simulink model "gm_sampleModel1971_sub"  (R2023a)
settings: Solver=VariableStepAuto  StartTime=0.0  StopTime=10.0  RelTol=1e-3
libraries: hdlsllib x1, simulink x1
settings Model: Creator=user1  LastModifiedBy=user1
settings OptimizationCC: BlockReduction=off  ConditionallyExecuteInputs=off
settings DebuggingCC: InheritedTsInSrcMsg=none

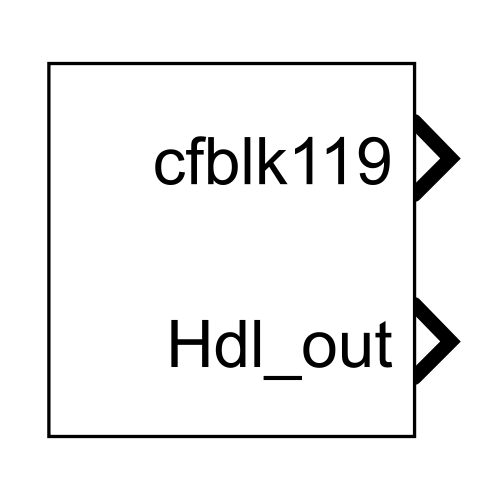
[thumbnail: Simulink's stored preview of the top-level diagram]
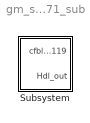
== system gm_sampleModel1971_sub ==
  Subsystem : Subsystem

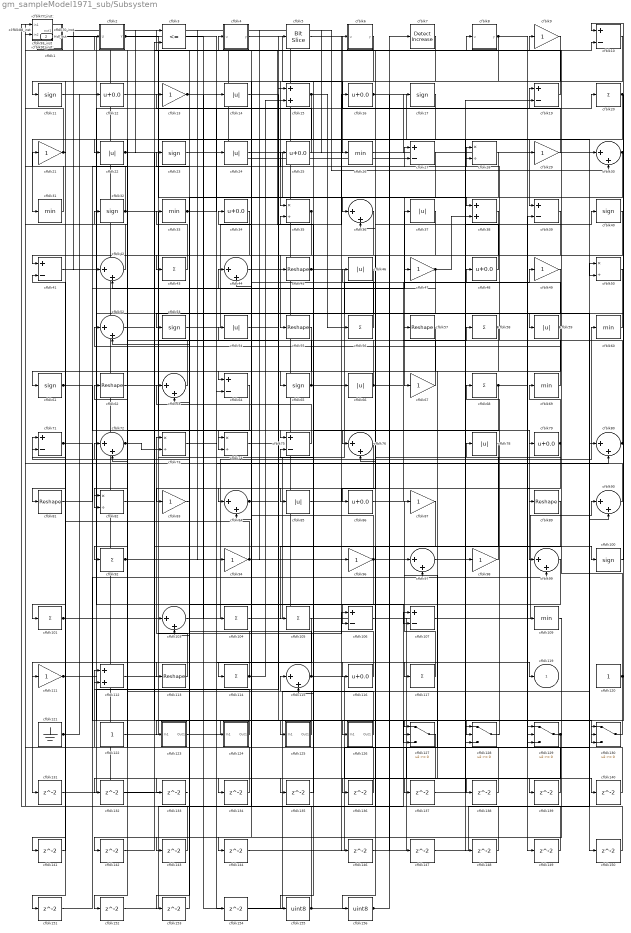
== system gm_sampleModel1971_sub/Subsystem ==
  cfblk1 : Subsystem  mask(Detect Fall Negative){vinit=double(0), InputProcessing=Elements as channels (sample based), OutDataTypeStr=uint8}
      mask prompts: vinit "Simulink:masks:InitialCondition_MP"; InputProcessing "Simulink:masks:InputProcessing_MP"; OutDataTypeStr "Simulink:masks:OutputDataType_MP"
      mask help: Simulink:masks:DetectFallNegative_MD
      mask init:
      | InputProcessing = 'Elements as channels (sample based)';
      | OutDataTypeStr = 'uint8';
      | vinit = double(0);
      mask TypeOptions InputProcessing: Simulink:masks:ColumnsAsChannelsFrameBased | Simulink:masks:ElementsAsChannelsSampleBased
      mask TypeOptions OutDataTypeStr: Simulink:masks:uint8 | Simulink:masks:boolean
      mask Display: fprintf('U < 0\n&  NOT\nU/z < 0')
  cfblk{10,19,27,39,41,64,71,75,106..107} (10 alike) : Sum  Inputs=+-  OutDataTypeStr=uint8
  cfblk{11,17,23,32,40,53,61,65,100} (9 alike) : Signum
  cfblk{20,43,56,58,68,92,101,104..105,114,117} (11 alike) : Sum  Inputs=+  OutDataTypeStr=uint8
  cfblk102_inst : Subsystem
  cfblk{30,36,42,44,52,63,72,76,80,84,90,97,99,103,115} (15 alike) : Sum  Inputs=|++  OutDataTypeStr=uint8
  cfblk108_inst : Subsystem
  cfblk{26,31,33,60,69,109} (6 alike) : MinMax  OutDataTypeStr=uint8
  cfblk110_inst : Subsystem
  cfblk{9,13,21,29,47,49,67,83,87,94,96,98,111} (13 alike) : Gain  OutDataTypeStr=uint8
  cfblk112 : Sum  OutDataTypeStr=uint8
  cfblk{45,55,57,62,81,89,113} (7 alike) : Reshape
  cfblk{12,16,25,34,48,79,86,116} (8 alike) : Bias  Bias=0.0  SaturateOnIntegerOverflow=off
  cfblk120 : Constant  OutDataTypeStr=uint8  SampleTime=-1
  cfblk121 : Ground
  cfblk122 : Constant  OutDataTypeStr=uint8  SampleTime=-1
  cfblk123 : Subsystem
  cfblk124 : Subsystem
  cfblk125 : Subsystem
  cfblk126 : Subsystem
  cfblk{127..130} (4 alike) : Switch  OutDataTypeStr=uint8  SaturateOnIntegerOverflow=off  InputSameDT=off
  cfblk{131..144,146..154} (23 alike) : Delay  SampleTime=1
  cfblk{14,22,24,37,46,54,59,66,78,85} (10 alike) : Abs  OutDataTypeStr=uint8  SaturateOnIntegerOverflow=off
  cfblk15 : Sum  OutDataTypeStr=uint8
  cfblk155 : DataTypeConversion  OutDataTypeStr=uint8  SaturateOnIntegerOverflow=off  RndMeth=Floor
  cfblk156 : DataTypeConversion  OutDataTypeStr=uint8  SaturateOnIntegerOverflow=off  RndMeth=Floor
  cfblk18_inst : Subsystem
  cfblk2 : Subsystem  mask(Detect Fall Nonpositive){vinit=double(0), InputProcessing=Elements as channels (sample based), OutDataTypeStr=uint8}
      mask prompts: vinit "Simulink:masks:InitialCondition_MP"; InputProcessing "Simulink:masks:InputProcessing_MP"; OutDataTypeStr "Simulink:masks:OutputDataType_MP"
      mask help: Simulink:masks:DetectFallNonpositive_MD
      mask init:
      | InputProcessing = 'Elements as channels (sample based)';
      | OutDataTypeStr = 'uint8';
      | vinit = double(0);
      mask TypeOptions InputProcessing: Simulink:masks:ColumnsAsChannelsFrameBased | Simulink:masks:ElementsAsChannelsSampleBased
      mask TypeOptions OutDataTypeStr: Simulink:masks:uint8 | Simulink:masks:boolean
      mask Display: fprintf('U <= 0\n&  NOT\nU/z <= 0')
  cfblk{28,35,50,73..74,82} (6 alike) : Product  Inputs=*/  OutDataTypeStr=uint8  RndMeth=Zero  SaturateOnIntegerOverflow=on
  cfblk3 : RelationalOperator  Operator=<=  OutDataTypeStr=boolean  InputSameDT=off
  cfblk38 : Sum  OutDataTypeStr=uint8
  cfblk4 : Subsystem  mask(Compare To Zero){relop=<=, OutDataTypeStr=uint8, ZeroCross=on}
      mask prompts: relop "Simulink:masks:Operator_MP"; OutDataTypeStr "Simulink:masks:OutputDataType_MP"; ZeroCross "Simulink:masks:EnableZerocrossingDetection_MP"
      mask help: Simulink:masks:CompareToZero_MD
      mask init:
      | OutDataTypeStr = 'uint8';
      | ZeroCross = 'on';
      | blkName = 'sampleModel1971_sub/Subsystem/cfblk4';
      | relop = '<=';
      | setValue = 'fixdt(0, 8)';
      mask TypeOptions relop: == | ~= | < | <= | >= | >
      mask TypeOptions OutDataTypeStr: Simulink:masks:uint8 | Simulink:masks:boolean
      mask Callback ZeroCross: sl('zeroCrossEnable', gcbh);
      mask Display: disp([relop,' 0'])
  cfblk5 : hdlsllib/Logic and Bit Operations/Bit Slice  lidx=7  ridx=0
  cfblk6 : Subsystem  mask(Compare To Zero){relop=<=, OutDataTypeStr=uint8, ZeroCross=on}
      mask prompts: relop "Simulink:masks:Operator_MP"; OutDataTypeStr "Simulink:masks:OutputDataType_MP"; ZeroCross "Simulink:masks:EnableZerocrossingDetection_MP"
      mask help: Simulink:masks:CompareToZero_MD
      mask init:
      | OutDataTypeStr = 'uint8';
      | ZeroCross = 'on';
      | blkName = 'sampleModel1971_sub/Subsystem/cfblk6';
      | relop = '<=';
      | setValue = 'fixdt(0, 8)';
      mask TypeOptions relop: == | ~= | < | <= | >= | >
      mask TypeOptions OutDataTypeStr: Simulink:masks:uint8 | Simulink:masks:boolean
      mask Callback ZeroCross: sl('zeroCrossEnable', gcbh);
      mask Display: disp([relop,' 0'])
  cfblk7 : simulink/Logic and Bit Operations/Detect Increase  vinit=0.0  OutDataTypeStr=uint8
      settings: LibrarySourceBlock=|
      | hdlsllib/Logic and Bit
      | Operations/Detect
      | Increase
  cfblk70_inst : Subsystem
  cfblk77_inst : Subsystem
  cfblk8 : Subsystem  mask(Compare To Zero){relop=<=, OutDataTypeStr=uint8, ZeroCross=on}
      mask prompts: relop "Simulink:masks:Operator_MP"; OutDataTypeStr "Simulink:masks:OutputDataType_MP"; ZeroCross "Simulink:masks:EnableZerocrossingDetection_MP"
      mask help: Simulink:masks:CompareToZero_MD
      mask init:
      | OutDataTypeStr = 'uint8';
      | ZeroCross = 'on';
      | blkName = 'sampleModel1971_sub/Subsystem/cfblk8';
      | relop = '<=';
      | setValue = 'fixdt(0, 8)';
      mask TypeOptions relop: == | ~= | < | <= | >= | >
      mask TypeOptions OutDataTypeStr: Simulink:masks:uint8 | Simulink:masks:boolean
      mask Callback ZeroCross: sl('zeroCrossEnable', gcbh);
      mask Display: disp([relop,' 0'])
  cfblk88_inst : Subsystem
  cfblk91_inst : Subsystem
  cfblk93_inst : Subsystem
  cfblk119 : Outport  OutDataTypeStr=uint8  SampleTime=1  VectorParamsAs1DForOutWhenUnconnected=off
  Hdl_out : Outport  Port=2  OutDataTypeStr=uint8  SampleTime=1
  wires:
  cfblk1/1(Y) -> cfblk75/1
  cfblk10/1 -> cfblk35/1
  cfblk100/1 -> cfblk10/1
  cfblk101/1 -> cfblk10/2, cfblk8/1(u)
  cfblk102_inst/1(out1) -> cfblk88_inst/2(in2), cfblk14/1
  cfblk103/1 -> cfblk60/1
  cfblk104/1 -> cfblk49/1
  cfblk105/1 -> cfblk131/1
  cfblk106/1 -> cfblk139/1
  cfblk107/1 -> cfblk90/1
  cfblk108_inst/1(out1) -> cfblk24/1
  cfblk109/1 -> cfblk142/1
  cfblk11/1 -> cfblk106/2
  cfblk110_inst/1(out1) -> cfblk96/1
  cfblk111/1 -> cfblk19/1, cfblk130/3
  cfblk112/1 -> cfblk94/1
  cfblk113/1 -> cfblk73/1
  cfblk114/1 -> cfblk72/1, cfblk15/2
  cfblk115/1 -> cfblk71/1, cfblk52/2, cfblk138/1
  cfblk116/1 -> cfblk35/2
  cfblk117/1 -> cfblk87/1
  cfblk12/1 -> cfblk38/1
  cfblk120/1 -> cfblk78/1, cfblk70_inst/2(in2), cfblk52/1, cfblk127/1
  cfblk121/1 -> cfblk91_inst/1(in1), cfblk12/1
  cfblk122/1 -> cfblk106/1
  cfblk123/1(Out1) -> cfblk128/2
  cfblk124/1(Out1) -> cfblk112/1
  cfblk125/1(Out1) -> cfblk62/1
  cfblk126/1(Out1) -> cfblk115/1
  cfblk127/1 -> cfblk152/1
  cfblk128/1 -> cfblk68/1
  cfblk129/1 -> cfblk134/1, cfblk133/1
  cfblk13/1 -> cfblk127/2, cfblk104/1
  cfblk130/1 -> cfblk123/1(In1)
  cfblk131/1 -> cfblk27/1
  cfblk132/1 -> cfblk28/1
  cfblk133/1 -> cfblk1/1(U)
  cfblk134/1 -> cfblk108_inst/2(in2)
  cfblk135/1 -> cfblk75/2
  cfblk136/1 -> cfblk72/2
  cfblk137/1 -> cfblk19/2
  cfblk138/1 -> cfblk77_inst/2(in2)
  cfblk139/1 -> cfblk97/1
  cfblk14/1 -> cfblk126/1(In1)
  cfblk140/1 -> cfblk112/2
  cfblk141/1 -> cfblk71/2
  cfblk142/1 -> cfblk103/1
  cfblk143/1 -> cfblk18_inst/1(in1)
  cfblk144/1 -> cfblk39/2
  cfblk146/1 -> cfblk90/2
  cfblk147/1 -> cfblk50/1
  cfblk148/1 -> cfblk93_inst/2(in2)
  cfblk149/1 -> cfblk44/2
  cfblk15/1 -> cfblk22/1, cfblk92/1, cfblk56/1
  cfblk150/1 -> cfblk36/2
  cfblk151/1 -> cfblk99/2
  cfblk152/1 -> cfblk107/1
  cfblk153/1 -> cfblk63/2
  cfblk154/1 -> cfblk80/1
  cfblk155/1 -> cfblk34/1, cfblk23/1
  cfblk156/1 -> Hdl_out/1, cfblk7/1
  cfblk16/1 -> cfblk129/2, cfblk148/1, cfblk147/1
  cfblk17/1 -> cfblk101/1
  cfblk18_inst/1(out1) -> cfblk30/2
  cfblk19/1 -> cfblk18_inst/2(in2)
  cfblk2/1(Y) -> cfblk39/1, cfblk50/2
  cfblk20/1 -> cfblk130/2, cfblk74/2, cfblk31/1
  cfblk21/1 -> cfblk91_inst/2(in2), cfblk61/1
  cfblk22/1 -> cfblk100/1, cfblk9/1
  cfblk23/1 -> cfblk116/1
  cfblk24/1 -> cfblk66/1
  cfblk25/1 -> cfblk4/1(u)
  cfblk26/1 -> cfblk17/1
  cfblk27/1 -> cfblk36/1
  cfblk28/1 -> cfblk67/1
  cfblk29/1 -> cfblk6/1(u)
  cfblk3/1 -> cfblk124/1(In1)
  cfblk30/1 -> cfblk85/1, cfblk83/1
  cfblk31/1 -> cfblk110_inst/1(in1)
  cfblk32/1 -> cfblk99/1, cfblk102_inst/2(in2)
  cfblk33/1 -> cfblk64/2, cfblk20/1
  cfblk34/1 -> cfblk43/1
  cfblk35/1 -> cfblk84/2, cfblk141/1
  cfblk36/1 -> cfblk114/1
  cfblk37/1 -> cfblk86/1
  cfblk38/1 -> cfblk82/2
  cfblk39/1 -> cfblk55/1
  cfblk4/1(y) -> cfblk26/1
  cfblk40/1 -> cfblk81/1
  cfblk41/1 -> cfblk59/1
  cfblk42/1 -> cfblk88_inst/1(in1)
  cfblk43/1 -> cfblk33/1
  cfblk44/1 -> cfblk5/1
  cfblk45/1 -> cfblk150/1, cfblk149/1
  cfblk46/1 -> cfblk65/1
  cfblk47/1 -> cfblk76/2, cfblk42/2, cfblk38/2, cfblk115/2
  cfblk48/1 -> cfblk77_inst/1(in1)
  cfblk49/1 -> cfblk153/1
  cfblk5/1 -> cfblk107/2
  cfblk50/1 -> cfblk53/1
  cfblk52/1 -> cfblk79/1
  cfblk53/1 -> cfblk16/1
  cfblk54/1 -> cfblk76/1
  cfblk55/1 -> cfblk111/1
  cfblk56/1 -> cfblk102_inst/1(in1)
  cfblk57/1 -> cfblk113/1
  cfblk58/1 -> cfblk84/1, cfblk137/1
  cfblk59/1 -> cfblk64/1, cfblk37/1, cfblk82/1
  cfblk6/1(y) -> cfblk144/1
  cfblk60/1 -> cfblk57/1
  cfblk61/1 -> cfblk74/1, cfblk151/1
  cfblk62/1 -> cfblk15/1
  cfblk63/1 -> cfblk93_inst/1(in1)
  cfblk64/1 -> cfblk132/1
  cfblk65/1 -> cfblk127/3, cfblk21/1
  cfblk66/1 -> cfblk54/1, cfblk48/1, cfblk46/1
  cfblk67/1 -> cfblk44/1
  cfblk68/1 -> cfblk129/1, cfblk135/1
  cfblk69/1 -> cfblk70_inst/1(in1)
  cfblk7/1 -> cfblk155/1
  cfblk70_inst/1(out1) -> cfblk109/1
  cfblk71/1 -> cfblk25/1, cfblk128/3
  cfblk72/1 -> cfblk32/1, cfblk73/2
  cfblk73/1 -> cfblk80/2
  cfblk74/1 -> cfblk45/1
  cfblk75/1 -> cfblk63/1
  cfblk76/1 -> cfblk143/1
  cfblk77_inst/1(out1) -> cfblk98/1
  cfblk78/1 -> cfblk156/1
  cfblk79/1 -> cfblk129/3, cfblk69/1
  cfblk8/1(y) -> cfblk130/1, cfblk11/1, cfblk140/1
  cfblk80/1 -> cfblk110_inst/2(in2), cfblk28/2
  cfblk81/1 -> cfblk47/1
  cfblk82/1 -> cfblk128/1
  cfblk83/1 -> cfblk3/1
  cfblk84/1 -> cfblk119/1, cfblk117/1
  cfblk85/1 -> cfblk89/1
  cfblk86/1 -> cfblk58/1
  cfblk87/1 -> cfblk136/1
  cfblk88_inst/1(out1) -> cfblk29/1
  cfblk89/1 -> cfblk105/1
  cfblk9/1 -> cfblk41/1
  cfblk90/1 -> cfblk108_inst/1(in1)
  cfblk91_inst/1(out1) -> cfblk30/1
  cfblk92/1 -> cfblk3/2, cfblk154/1
  cfblk93_inst/1(out1) -> cfblk42/1, cfblk27/2
  cfblk94/1 -> cfblk97/2, cfblk41/2, cfblk146/1
  cfblk96/1 -> cfblk13/1, cfblk125/1(In1)
  cfblk97/1 -> cfblk40/1
  cfblk98/1 -> cfblk2/1(U)
  cfblk99/1 -> cfblk103/2

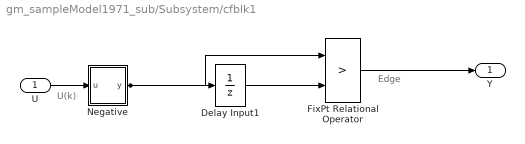
== system gm_sampleModel1971_sub/Subsystem/cfblk1 ==
  note: U(k)
  note: Edge
  U : Inport  OutDataTypeStr=uint8  SampleTime=1
  Delay Input1 : UnitDelay  Description=Store in Global RAM  DisableCoverage=on  InitialCondition=vinit  SampleTime=-1  HasFrameUpgradeWarning=on
  FixPt Relational Operator : RelationalOperator  Operator=>  OutDataTypeStr=fixdt(0, 8)  ZeroCross=off  InputSameDT=off
  Negative : Subsystem  mask(Compare To Zero){relop=<, OutDataTypeStr=boolean, ZeroCross=off}
      mask prompts: relop "Simulink:masks:Operator_MP"; OutDataTypeStr "Simulink:masks:OutputDataType_MP"; ZeroCross "Simulink:masks:EnableZerocrossingDetection_MP"
      mask help: Simulink:masks:CompareToZero_MD
      mask init:
      | OutDataTypeStr = 'boolean';
      | ZeroCross = 'off';
      | blkName = 'sampleModel1971_sub/Subsystem/cfblk1/Negative';
      | relop = '<';
      | setValue = 'boolean';
      mask TypeOptions relop: == | ~= | < | <= | >= | >
      mask TypeOptions OutDataTypeStr: Simulink:masks:uint8 | Simulink:masks:boolean
      mask Callback ZeroCross: sl('zeroCrossEnable', gcbh);
      mask Display: disp([relop,' 0'])
  Y : Outport  SampleTime=1
  wires:
  U/1 -> Negative/1(u)
  Delay Input1/1 -> FixPt Relational Operator/2
  FixPt Relational Operator/1 -> Y/1
  Negative/1(y) -> FixPt Relational Operator/1, Delay Input1/1

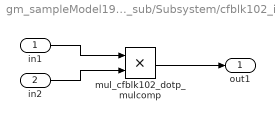
== system gm_sampleModel1971_sub/Subsystem/cfblk102_inst ==
  in1 : Inport  OutDataTypeStr=uint8  SampleTime=1
  in2 : Inport  Port=2  OutDataTypeStr=uint8  SampleTime=1
  mul_cfblk102_dotp_mulcomp : Product  Inputs=**  OutDataTypeStr=uint8  SampleTime=1
  out1 : Outport  OutDataTypeStr=uint8  SampleTime=1
  wires:
  in1/1 -> mul_cfblk102_dotp_mulcomp/1
  in2/1 -> mul_cfblk102_dotp_mulcomp/2
  mul_cfblk102_dotp_mulcomp/1 -> out1/1

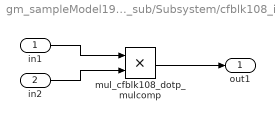
== system gm_sampleModel1971_sub/Subsystem/cfblk108_inst ==
  in1 : Inport  OutDataTypeStr=uint8  SampleTime=1
  in2 : Inport  Port=2  OutDataTypeStr=uint8  SampleTime=1
  mul_cfblk108_dotp_mulcomp : Product  Inputs=**  OutDataTypeStr=uint8  SampleTime=1
  out1 : Outport  OutDataTypeStr=uint8  SampleTime=1
  wires:
  in1/1 -> mul_cfblk108_dotp_mulcomp/1
  in2/1 -> mul_cfblk108_dotp_mulcomp/2
  mul_cfblk108_dotp_mulcomp/1 -> out1/1

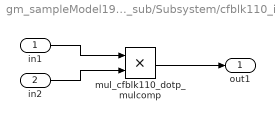
== system gm_sampleModel1971_sub/Subsystem/cfblk110_inst ==
  in1 : Inport  OutDataTypeStr=uint8  SampleTime=1
  in2 : Inport  Port=2  OutDataTypeStr=uint8  SampleTime=1
  mul_cfblk110_dotp_mulcomp : Product  Inputs=**  OutDataTypeStr=uint8  SampleTime=1
  out1 : Outport  OutDataTypeStr=uint8  SampleTime=1
  wires:
  in1/1 -> mul_cfblk110_dotp_mulcomp/1
  in2/1 -> mul_cfblk110_dotp_mulcomp/2
  mul_cfblk110_dotp_mulcomp/1 -> out1/1

== system gm_sampleModel1971_sub/Subsystem/cfblk123 ==
  In1 : Inport  OutDataTypeStr=uint8  PortDimensions=1  SampleTime=1
  Out1 : Outport  SampleTime=1
  wires:
  In1/1 -> Out1/1

== system gm_sampleModel1971_sub/Subsystem/cfblk124 ==
  In1 : Inport  OutDataTypeStr=boolean  PortDimensions=1  SampleTime=1
  Out1 : Outport  SampleTime=1
  wires:
  In1/1 -> Out1/1

== system gm_sampleModel1971_sub/Subsystem/cfblk125 ==
  In1 : Inport  OutDataTypeStr=uint8  PortDimensions=1  SampleTime=1
  Out1 : Outport  SampleTime=1
  wires:
  In1/1 -> Out1/1

== system gm_sampleModel1971_sub/Subsystem/cfblk126 ==
  In1 : Inport  OutDataTypeStr=uint8  PortDimensions=1  SampleTime=1
  Out1 : Outport  SampleTime=1
  wires:
  In1/1 -> Out1/1

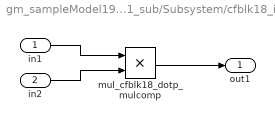
== system gm_sampleModel1971_sub/Subsystem/cfblk18_inst ==
  in1 : Inport  OutDataTypeStr=uint8  SampleTime=1
  in2 : Inport  Port=2  OutDataTypeStr=uint8  SampleTime=1
  mul_cfblk18_dotp_mulcomp : Product  Inputs=**  OutDataTypeStr=uint8  SampleTime=1
  out1 : Outport  OutDataTypeStr=uint8  SampleTime=1
  wires:
  in1/1 -> mul_cfblk18_dotp_mulcomp/1
  in2/1 -> mul_cfblk18_dotp_mulcomp/2
  mul_cfblk18_dotp_mulcomp/1 -> out1/1

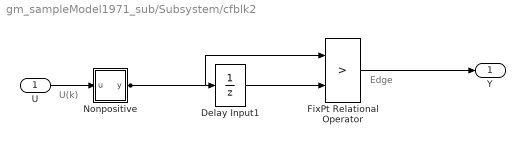
== system gm_sampleModel1971_sub/Subsystem/cfblk2 ==
  note: U(k)
  note: Edge
  U : Inport  OutDataTypeStr=uint8  SampleTime=1
  Delay Input1 : UnitDelay  Description=Store in Global RAM  DisableCoverage=on  InitialCondition=vinit  SampleTime=-1  HasFrameUpgradeWarning=on
  FixPt Relational Operator : RelationalOperator  Operator=>  OutDataTypeStr=fixdt(0, 8)  ZeroCross=off  InputSameDT=off
  Nonpositive : Subsystem  mask(Compare To Zero){relop=<=, OutDataTypeStr=boolean, ZeroCross=off}
      mask prompts: relop "Simulink:masks:Operator_MP"; OutDataTypeStr "Simulink:masks:OutputDataType_MP"; ZeroCross "Simulink:masks:EnableZerocrossingDetection_MP"
      mask help: Simulink:masks:CompareToZero_MD
      mask init:
      | OutDataTypeStr = 'boolean';
      | ZeroCross = 'off';
      | blkName = 'sampleModel1971_sub/Subsystem/cfblk2/Nonpositive';
      | relop = '<=';
      | setValue = 'boolean';
      mask TypeOptions relop: == | ~= | < | <= | >= | >
      mask TypeOptions OutDataTypeStr: Simulink:masks:uint8 | Simulink:masks:boolean
      mask Callback ZeroCross: sl('zeroCrossEnable', gcbh);
      mask Display: disp([relop,' 0'])
  Y : Outport  SampleTime=1
  wires:
  U/1 -> Nonpositive/1(u)
  Delay Input1/1 -> FixPt Relational Operator/2
  FixPt Relational Operator/1 -> Y/1
  Nonpositive/1(y) -> FixPt Relational Operator/1, Delay Input1/1

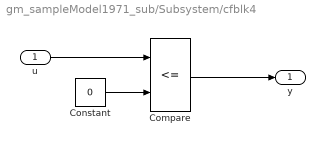
== system gm_sampleModel1971_sub/Subsystem/cfblk4 ==
  u : Inport  OutDataTypeStr=uint8  SampleTime=1
  Compare : RelationalOperator  Operator=<=  OutDataTypeStr=fixdt(0, 8)
  Constant : Constant  DisableCoverage=on  Value=0  OutDataTypeStr=Inherit: Inherit via back propagation  SampleTime=-1  PreserveConstantTs=on
  y : Outport  SampleTime=1
  wires:
  u/1 -> Compare/1
  Compare/1 -> y/1
  Constant/1 -> Compare/2

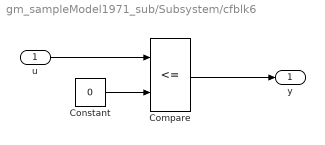
== system gm_sampleModel1971_sub/Subsystem/cfblk6 ==
  u : Inport  OutDataTypeStr=uint8  SampleTime=1
  Compare : RelationalOperator  Operator=<=  OutDataTypeStr=fixdt(0, 8)
  Constant : Constant  DisableCoverage=on  Value=0  OutDataTypeStr=Inherit: Inherit via back propagation  SampleTime=-1  PreserveConstantTs=on
  y : Outport  SampleTime=1
  wires:
  u/1 -> Compare/1
  Compare/1 -> y/1
  Constant/1 -> Compare/2

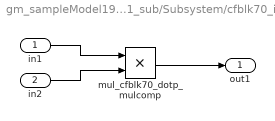
== system gm_sampleModel1971_sub/Subsystem/cfblk70_inst ==
  in1 : Inport  OutDataTypeStr=uint8  SampleTime=1
  in2 : Inport  Port=2  OutDataTypeStr=uint8  SampleTime=1
  mul_cfblk70_dotp_mulcomp : Product  Inputs=**  OutDataTypeStr=uint8  SampleTime=1
  out1 : Outport  OutDataTypeStr=uint8  SampleTime=1
  wires:
  in1/1 -> mul_cfblk70_dotp_mulcomp/1
  in2/1 -> mul_cfblk70_dotp_mulcomp/2
  mul_cfblk70_dotp_mulcomp/1 -> out1/1

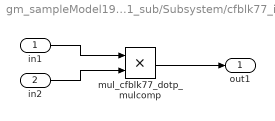
== system gm_sampleModel1971_sub/Subsystem/cfblk77_inst ==
  in1 : Inport  OutDataTypeStr=uint8  SampleTime=1
  in2 : Inport  Port=2  OutDataTypeStr=uint8  SampleTime=1
  mul_cfblk77_dotp_mulcomp : Product  Inputs=**  OutDataTypeStr=uint8  SampleTime=1
  out1 : Outport  OutDataTypeStr=uint8  SampleTime=1
  wires:
  in1/1 -> mul_cfblk77_dotp_mulcomp/1
  in2/1 -> mul_cfblk77_dotp_mulcomp/2
  mul_cfblk77_dotp_mulcomp/1 -> out1/1

== system gm_sampleModel1971_sub/Subsystem/cfblk8 ==
  u : Inport  OutDataTypeStr=uint8  SampleTime=1
  Compare : RelationalOperator  Operator=<=  OutDataTypeStr=fixdt(0, 8)
  Constant : Constant  DisableCoverage=on  Value=0  OutDataTypeStr=Inherit: Inherit via back propagation  SampleTime=-1  PreserveConstantTs=on
  y : Outport  SampleTime=1
  wires:
  u/1 -> Compare/1
  Compare/1 -> y/1
  Constant/1 -> Compare/2

== system gm_sampleModel1971_sub/Subsystem/cfblk88_inst ==
  in1 : Inport  OutDataTypeStr=uint8  SampleTime=1
  in2 : Inport  Port=2  OutDataTypeStr=uint8  SampleTime=1
  mul_cfblk88_dotp_mulcomp : Product  Inputs=**  OutDataTypeStr=uint8  SampleTime=1
  out1 : Outport  OutDataTypeStr=uint8  SampleTime=1
  wires:
  in1/1 -> mul_cfblk88_dotp_mulcomp/1
  in2/1 -> mul_cfblk88_dotp_mulcomp/2
  mul_cfblk88_dotp_mulcomp/1 -> out1/1

== system gm_sampleModel1971_sub/Subsystem/cfblk91_inst ==
  in1 : Inport  OutDataTypeStr=uint8  SampleTime=1
  in2 : Inport  Port=2  OutDataTypeStr=uint8  SampleTime=1
  mul_cfblk91_dotp_mulcomp : Product  Inputs=**  OutDataTypeStr=uint8  SampleTime=1
  out1 : Outport  OutDataTypeStr=uint8  SampleTime=1
  wires:
  in1/1 -> mul_cfblk91_dotp_mulcomp/1
  in2/1 -> mul_cfblk91_dotp_mulcomp/2
  mul_cfblk91_dotp_mulcomp/1 -> out1/1

== system gm_sampleModel1971_sub/Subsystem/cfblk93_inst ==
  in1 : Inport  OutDataTypeStr=uint8  SampleTime=1
  in2 : Inport  Port=2  OutDataTypeStr=uint8  SampleTime=1
  mul_cfblk93_dotp_mulcomp : Product  Inputs=**  OutDataTypeStr=uint8  SampleTime=1
  out1 : Outport  OutDataTypeStr=uint8  SampleTime=1
  wires:
  in1/1 -> mul_cfblk93_dotp_mulcomp/1
  in2/1 -> mul_cfblk93_dotp_mulcomp/2
  mul_cfblk93_dotp_mulcomp/1 -> out1/1

== system gm_sampleModel1971_sub/Subsystem/cfblk1/Negative ==
  u : Inport  OutDataTypeStr=uint8  SampleTime=1
  Compare : RelationalOperator  Operator=<  OutDataTypeStr=boolean  ZeroCross=off
  Constant : Constant  DisableCoverage=on  Value=0  OutDataTypeStr=Inherit: Inherit via back propagation  SampleTime=-1  PreserveConstantTs=on
  y : Outport  SampleTime=1
  wires:
  u/1 -> Compare/1
  Compare/1 -> y/1
  Constant/1 -> Compare/2

== system gm_sampleModel1971_sub/Subsystem/cfblk2/Nonpositive ==
  u : Inport  OutDataTypeStr=uint8  SampleTime=1
  Compare : RelationalOperator  Operator=<=  OutDataTypeStr=boolean  ZeroCross=off
  Constant : Constant  DisableCoverage=on  Value=0  OutDataTypeStr=Inherit: Inherit via back propagation  SampleTime=-1  PreserveConstantTs=on
  y : Outport  SampleTime=1
  wires:
  u/1 -> Compare/1
  Compare/1 -> y/1
  Constant/1 -> Compare/2
